simulink model "Simulink1"  (R2016a)
settings: Solver=VariableStepAuto  StartTime=0.0  StopTime=Tsim  RelTol=1e-3
values from neighbouring files (symbols this model uses):
  F1 = 85005.9    [Script.m]
  F2 = 90000    [Script.m]
  F3 = 94986.8    [Script.m]
  F4 = 100000    [Script.m]
  F5 = 115015.9    [Script.m]
  F6 = 120000    [Script.m]
  Te = 1/320000    (= 3.125e-06)    [Script.m]
  Ts = Te/100    (= 3.125e-08)    [Script.m]
settings Model: Creator=ferrandi  LastModifiedBy=ferrandi

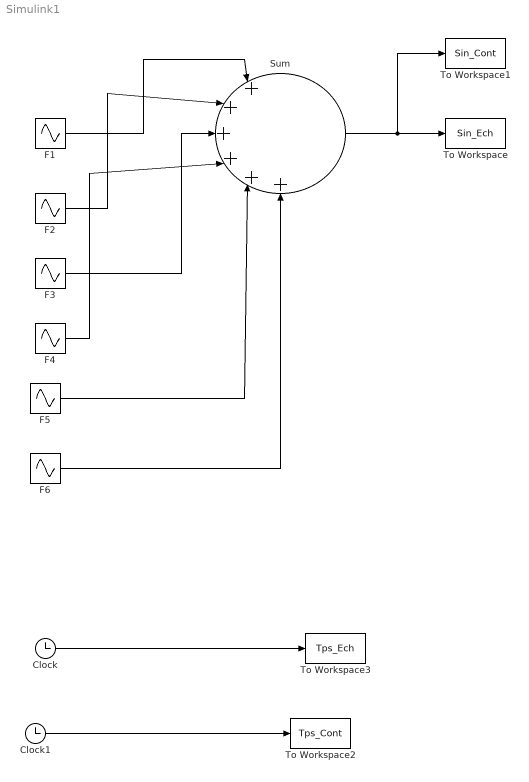
== system Simulink1 ==
  Clock : Clock
  Clock1 : Clock
  F1 : Sin  Amplitude=5  Frequency=F1*2*pi  SampleTime=0
  F2 : Sin  Amplitude=5  Frequency=F2*2*pi  SampleTime=0
  F3 : Sin  Amplitude=5  Frequency=F3*2*pi  SampleTime=0
  F4 : Sin  Amplitude=5  Frequency=F4*2*pi  SampleTime=0
  F5 : Sin  Amplitude=5  Frequency=F5*2*pi  SampleTime=0
  F6 : Sin  Amplitude=5  Frequency=F6*2*pi  SampleTime=0
  Sum : Sum  Inputs=|++++++
  To Workspace : ToWorkspace  VariableName=Sin_Ech  SaveFormat=Timeseries  SampleTime=Te
  To Workspace1 : ToWorkspace  VariableName=Sin_Cont  SaveFormat=Timeseries  SampleTime=Ts
  To Workspace2 : ToWorkspace  VariableName=Tps_Cont  SaveFormat=Timeseries  SampleTime=Ts
  To Workspace3 : ToWorkspace  VariableName=Tps_Ech  SaveFormat=Timeseries  SampleTime=Te
  wires:
  Clock1/1 -> To Workspace2/1
  Clock/1 -> To Workspace3/1
  F1/1 -> Sum/1
  Sum/1 -> To Workspace1/1, To Workspace/1
  F2/1 -> Sum/2
  F3/1 -> Sum/3
  F4/1 -> Sum/4
  F5/1 -> Sum/5
  F6/1 -> Sum/6
